simulink model "quantif"  (Simulink 7.3)
settings: Solver=ode45  StartTime=0.0  StopTime=10.0  RelTol=1e-3
values from neighbouring files (symbols this model uses):
  A0 = 1.5    [Init_quantif.m]
  f0 = 1    [Init_quantif.m]
  fe = 15    [Init_quantif.m]
libraries: commnoisgen2 x1, dspstat3 x1, simulink x1
settings Model: Creator=conteville  LastModifiedBy=conteville

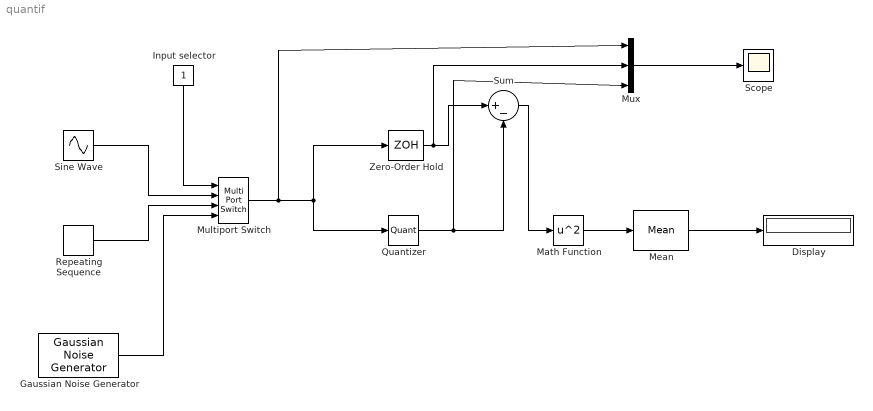
== system quantif ==
  Display : Display
  Gaussian Noise Generator : commnoisgen2/Gaussian Noise Generator  SystemSampleTime=-1  m=0  d=1  s=41  Ts=1  frameBased=off  sampPerFrame=1  orient=off  outDataType=double
  Input selector : Constant
  Math Function : Math  Operator=square  SaturateOnIntegerOverflow=on
  Mean : dspstat3/Mean  DialogController=dspDDGCreate  DialogControllerArgs=DataTag0  run=off  reset_popup=None  directionMode=Each column  dimension=1  treatSBRowAsCol=on  roiEnable=off  roiType=Rectangles  roiPortion=Entire ROI  roiOutput=Individual statistics for each ROI  roiFlag=off  roundingMode=Floor  overflowMode=off
  Multiport Switch : MultiPortSwitch  OutDataType=fixdt(1, 16)  OutScaling=2^0
  Mux : Mux  Inputs=3
  Quantizer : Quantizer  QuantizationInterval=q
  Repeating Sequence : simulink/Sources/Repeating Sequence  SystemSampleTime=-1  rep_seq_t=[0 2]  rep_seq_y=[0 2]
  Scope : Scope
  Sine Wave : Sin  Amplitude=A0  Bias=0  Frequency=2*pi*f0  Phase=0  Samples=10  SampleTime=0  Offset=0
  Sum : Sum  Inputs=|+-  OutDataType=fixdt(1, 16)  OutScaling=2^0
  Zero-Order Hold : ZeroOrderHold  SampleTime=1/fe
  wires:
  Input selector/1 -> Multiport Switch/1
  Sine Wave/1 -> Multiport Switch/2
  Repeating Sequence/1 -> Multiport Switch/3
  Gaussian Noise Generator/1 -> Multiport Switch/4
  Multiport Switch/1 -> Zero-Order Hold/1, Quantizer/1, Mux/1
  Zero-Order Hold/1 -> Sum/1, Mux/2
  Quantizer/1 -> Sum/2, Mux/3
  Sum/1 -> Math Function/1
  Math Function/1 -> Mean/1
  Mean/1 -> Display/1
  Mux/1 -> Scope/1
